simulink model "quizq2b"  (R2013b)
settings: Solver=ode4  StartTime=0.0  StopTime=25  RelTol=1e-3
undefined symbols (not defined in the file): A, B, C, D
settings Model: Creator=makha  LastModifiedBy=Zeerak Nadeem Wyne
settings DataIOCC: LimitDataPoints=off  SaveFormat=Dataset
settings OptimizationCC: LifeSpan=auto  SimCompilerOptimization=off
settings DebuggingCC: UnderspecifiedInitializationDetection=Simplified  MergeDetectMultiDrivingBlocksExec=error  SolverPrmCheckMsg=none  FcnCallInpInsideContextMsg=error  FrameProcessingCompatibilityMsg=error  LibraryContextMissingDiagnostic=warning  SFUnexpectedBacktrackingDiag=error  SFNoUnconditionalDefaultTransitionDiag=error
settings HardwareCC: ProdBitPerPointer=64  ProdLargestAtomicFloat=Float  ProdIntDivRoundTo=Zero  ProdEndianess=LittleEndian  ProdWordSize=64  ProdHWDeviceType=Intel->x86-64 (Windows64)
settings ModelReferenceCC: PropagateSignalLabelsOutOfModel=on
settings SFSimCC: SimUseLocalCustomCode=on
settings RTWCC: RTWUseLocalCustomCode=on  RTWCompilerOptimization=off
settings GRTTargetCC: CodeReplacementLibrary=None  GeneratePreprocessorConditionals=Use local settings  CPPClassGenCompliant=on

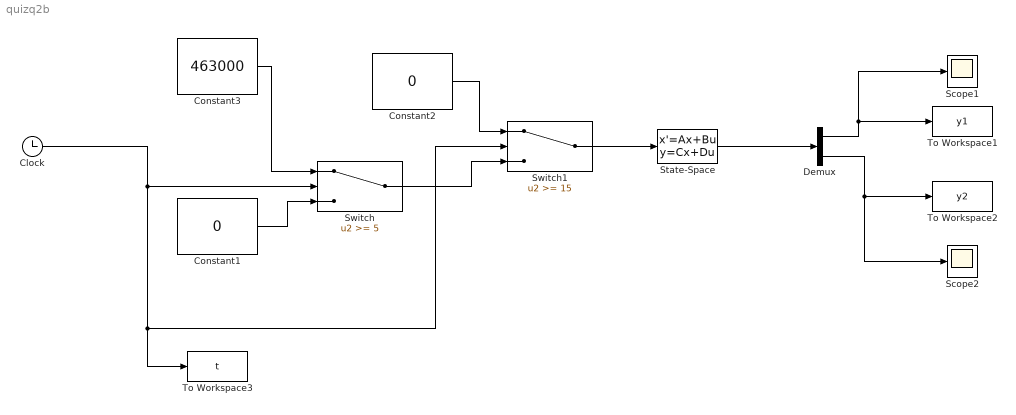
== system quizq2b ==
  Clock : Clock
      settings: Decimation=1000
  Constant1 : Constant  Value=0
  Constant2 : Constant  Value=0
  Constant3 : Constant  Value=463000
  Demux : Demux  Outputs=2
  Scope1 : Scope
  Scope2 : Scope
      settings: SaveName=ScopeData2
  State-Space : StateSpace  A=A  B=B  C=C  D=D
  Switch : Switch  Threshold=5  SaturateOnIntegerOverflow=off  InputSameDT=off
  Switch1 : Switch  Threshold=15  SaturateOnIntegerOverflow=off  InputSameDT=off
  To Workspace1 : ToWorkspace  VariableName=y1  SampleTime=-1
  To Workspace2 : ToWorkspace  VariableName=y2  SampleTime=-1
  To Workspace3 : ToWorkspace  VariableName=t  SampleTime=-1
  wires:
  Demux/1 -> Scope1/1, To Workspace1/1
  Demux/2 -> To Workspace2/1, Scope2/1
  State-Space/1 -> Demux/1
  Switch1/1 -> State-Space/1
  Clock/1 -> To Workspace3/1, Switch1/2, Switch/2
  Switch/1 -> Switch1/3
  Constant1/1 -> Switch/3
  Constant2/1 -> Switch1/1
  Constant3/1 -> Switch/1
